simulink model "Three_ph_VSI_R2017a"  (R2020b)
settings: Solver=ode23tb  StartTime=0.0  StopTime=0.5  MaxStep=1e-6  RelTol=1e-3  EnableMultiTasking=on
libraries: powerlib x16, simulink x1
settings Model: Creator=shaheb  LastModifiedBy=HP
settings DataIOCC: LimitDataPoints=on  SaveFormat=Array  SignalLoggingSaveFormat=ModelDataLogs  ReturnWorkspaceOutputs=off
settings OptimizationCC: ExpressionDepthLimit=2147483647  LifeSpan=inf
settings DebuggingCC: UnderspecifiedInitializationDetection=Classic  MergeDetectMultiDrivingBlocksExec=none  SolverPrmCheckMsg=warning  FcnCallInpInsideContextMsg=warning  StateNameClashWarn=warning  SFUnexpectedBacktrackingDiag=warning  SFNoUnconditionalDefaultTransitionDiag=warning  ArithmeticOperatorsInVariantConditions=warning
settings HardwareCC: ProdBitPerPointer=32  ProdBitPerSizeT=32  ProdBitPerPtrDiffT=32  ProdLargestAtomicFloat=None  ProdIntDivRoundTo=Undefined  ProdEndianess=Unspecified  ProdWordSize=32  ProdHWDeviceType=32-bit Generic
settings ModelReferenceCC: PropagateSignalLabelsOutOfModel=off
settings SFSimCC: SimUseLocalCustomCode=off  CustomCodeUndefinedFunction=UseInterfaceOnly
settings RTWCC: RTWUseLocalCustomCode=off
settings CodeAppCC: StateflowObjectComments=on
settings GRTTargetCC: TargetLangStandard=C89/C90 (ANSI)  CombineOutputUpdateFcns=off  GRTInterface=on
settings ConfigComp: CovMetricSettings=dw  CovSaveCumulativeToWorkspaceVar=on  CovSaveSingleToWorkspaceVar=on  CovExternalEMLEnable=off
settings SimscapeCC: SimscapeNormalizeSystem=off

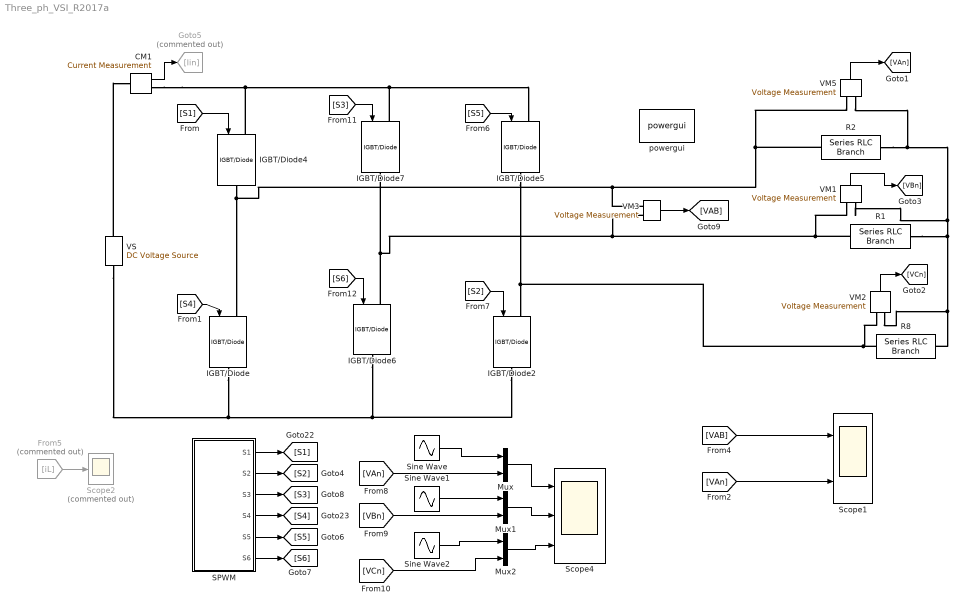
== system Three_ph_VSI_R2017a ==
  CM1 : powerlib/Measurements/Current Measurement  PhasorSimulation=off  OutputType=Complex  PSBequivalent=0
  From5 : From  Commented=on  GotoTag=iL
  Goto5 : Goto  Commented=on  GotoTag=Iin
  IGBT/Diode{,2,4..7} (6 alike) : powerlib/Power Electronics/IGBT//Diode  Ron=20e-3  Rs=1e5  Cs=inf  Measurements=off
  Mux : Mux  Inputs=2
  Mux1 : Mux  Inputs=2
  Mux2 : Mux  Inputs=2
  R1 : powerlib/Elements/Series RLC Branch  LConnTagsString=__new0  RConnTagsString=__new0  BranchType=RL  Resistance=40  Inductance=20e-3  SetiL0=off  InitialCurrent=0  Capacitance=500e-6  Setx0=off  InitialVoltage=0  Measurements=None
  R2 : powerlib/Elements/Series RLC Branch  LConnTagsString=__new0  RConnTagsString=__new0  BranchType=RL  Resistance=40  Inductance=20e-3  SetiL0=off  InitialCurrent=0  Capacitance=500e-6  Setx0=off  InitialVoltage=0  Measurements=None
  R8 : powerlib/Elements/Series RLC Branch  LConnTagsString=__new0  RConnTagsString=__new0  BranchType=RL  Resistance=40  Inductance=20e-3  SetiL0=off  InitialCurrent=0  Capacitance=500e-6  Setx0=off  InitialVoltage=0  Measurements=None
  SPWM : Subsystem
  Scope1 : Scope  NumInputPorts=2
  Scope2 : Scope  Commented=on
  Scope4 : Scope  NumInputPorts=3
  Sine Wave : Sin  Amplitude=230*sqrt(2)  Frequency=2*pi*50  SampleTime=0
  Sine Wave1 : Sin  Amplitude=230*sqrt(2)  Frequency=2*pi*50  Phase=-(2*pi/3)  SampleTime=0
  Sine Wave2 : Sin  Amplitude=230*sqrt(2)  Frequency=2*pi*50  Phase=+(2*pi/3)  SampleTime=0
  VM{1..3,5} (4 alike) : powerlib/Measurements/Voltage Measurement  PhasorSimulation=off  OutputType=Complex  PSBequivalent=0
  VS : powerlib/Electrical Sources/DC Voltage Source  Amplitude=700  Measurements=None
  powergui : powerlib/powergui  Priority=1  SimulationMode=Discrete  SampleTime=1e-6  frequency=60  Iterations=50  frequencyindice=0  Pbase=100e6  ErrMax=1e-4  UnitsV=kV  UnitsW=MW  buscounter=0  FunctionMessages=off  echomessages=off  EnableUseOfTLC=off  CurrentSourceSwitches=off  DisableSnubberDevices=off  DisableRonSwitches=off  DisableVfSwitches=off  DisplayEquations=off  AutomaticDiscreteSolvers=off  SolverType=Tustin  Interpol=off  ExternalGateDelay=off  methode=off  Ts=10  x0status=blocks  SPID=off  SwTol=0  HookPort=off  NonlinearTolerance=1e-4  nMaxIteration=100  ContinueOnMaxIteration=off  RestoreLinks=warning  ResistiveCurrentMeasurement=off  Frange=[0:2:500]  Ylog=off  Xlog=on  ShowGrid=off  save=off  variable=ZData  structure=vo  ZoomFFT=off  StartTime=0.2  cycles=10  DisplayStyle=1  fundamental=50  FreqAxis=on  MaxFrequency=20000  frequencyindicesteady=1  RmsSteady=1  display=off
  wires:
  [VAB] -> Scope1/1
  From5/1 -> Scope2/1
  SPWM/1(S1) -> [S1]
  SPWM/4(S4) -> [S4]
  VM2/1 -> [VCn]
  SPWM/6(S6) -> [S6]
  SPWM/5(S5) -> [S5]
  SPWM/3(S3) -> [S3]
  SPWM/2(S2) -> [S2]
  Sine Wave/1 -> Mux/1
  [VAn] -> Mux/2
  Mux/1 -> Scope4/1
  Sine Wave1/1 -> Mux1/1
  [VBn] -> Mux1/2
  Mux1/1 -> Scope4/2
  Sine Wave2/1 -> Mux2/1
  [VCn] -> Mux2/2
  Mux2/1 -> Scope4/3
  [S1] -> IGBT/Diode4/1
  [S4] -> IGBT/Diode/1
  CM1/1 -> Goto5/1
  [S5] -> IGBT/Diode5/1
  [S2] -> IGBT/Diode2/1
  [S3] -> IGBT/Diode7/1
  [S6] -> IGBT/Diode6/1
  VM5/1 -> [VAn]
  VM1/1 -> [VBn]
  VM3/1 -> [VAB]
  [VAn] -> Scope1/2
  connections:
  R2/LConn1 -- VM1/LConn2 -- R1/LConn1 -- VM2/LConn2 -- R8/LConn1 -- VM5/LConn2
  CM1/RConn1 -- IGBT/Diode4/LConn1 -- IGBT/Diode7/LConn1 -- IGBT/Diode5/LConn1
  IGBT/Diode7/RConn1 -- VM3/LConn2 -- R1/RConn1 -- VM1/LConn1 -- IGBT/Diode6/LConn1
  VS/LConn1 -- IGBT/Diode2/RConn1 -- IGBT/Diode6/RConn1 -- IGBT/Diode/RConn1
  IGBT/Diode4/RConn1 -- VM5/LConn1 -- R2/RConn1 -- VM3/LConn1 -- IGBT/Diode/LConn1
  IGBT/Diode5/RConn1 -- VM2/LConn1 -- R8/RConn1 -- IGBT/Diode2/LConn1
  VS/RConn1 -- CM1/LConn1

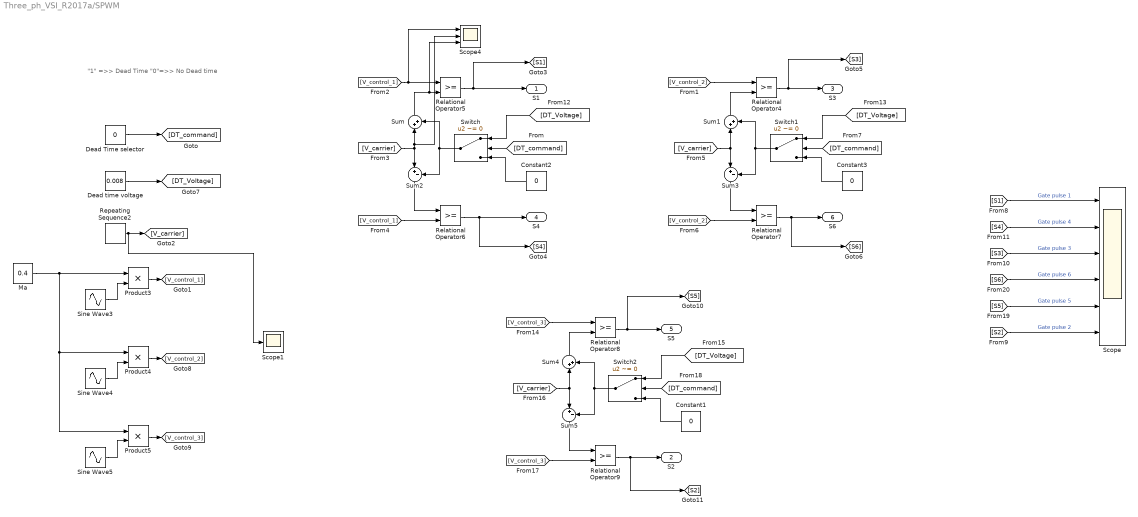
== system Three_ph_VSI_R2017a/SPWM ==
  note: "1" =>> Dead Time
      | "0"=>> No Dead time
  Constant1 : Constant  Value=0
  Constant2 : Constant  Value=0
  Constant3 : Constant  Value=0
  Dead Time selector : Constant  Value=0
  Dead time voltage : Constant  Value=0.008
  Ma : Constant  Value=0.4
  Product3 : Product
  Product4 : Product
  Product5 : Product
  Relational Operator{4..9} (6 alike) : RelationalOperator  OutDataTypeStr=boolean  RndMeth=Nearest
  Repeating Sequence2 : simulink/Sources/Repeating Sequence  rep_seq_t=[0 1/4 1/2 3/4 1/1]*1/(15*1000)  rep_seq_y=[0 1 0 -1 0]
  Scope : Scope  NumInputPorts=6
  Scope1 : Scope
  Scope4 : Scope  NumInputPorts=3
  Sine Wave3 : Sin  Frequency=2*pi*50  SampleTime=0
  Sine Wave4 : Sin  Frequency=2*pi*50  Phase=-(2*pi/3)  SampleTime=0
  Sine Wave5 : Sin  Frequency=2*pi*50  Phase=+(2*pi/3)  SampleTime=0
  Sum : Sum  Inputs=|++
  Sum1 : Sum  Inputs=|++
  Sum2 : Sum  Inputs=|+-
  Sum3 : Sum  Inputs=|+-
  Sum4 : Sum  Inputs=|++
  Sum5 : Sum  Inputs=|+-
  Switch : Switch  Criteria=u2 ~= 0
  Switch1 : Switch  Criteria=u2 ~= 0
  Switch2 : Switch  Criteria=u2 ~= 0
  S1 : Outport
  S2 : Outport  Port=2
  S3 : Outport  Port=3
  S4 : Outport  Port=4
  S5 : Outport  Port=5
  S6 : Outport  Port=6
  wires:
  Relational Operator6/1 -> S4/1, [S4]
  Constant2/1 -> Switch/3
  [V_control_1] -> Scope4/1, Relational Operator5/1
  Sum/1 -> Scope4/3, Relational Operator5/2
  [V_carrier] -> Scope4/2, Sum/1, Sum2/1
  Sine Wave3/1 -> Product3/2
  Dead time voltage/1 -> [DT_Voltage]
  Relational Operator5/1 -> [S1], S1/1
  [DT_Voltage] -> Switch/1
  Relational Operator4/1 -> S3/1, [S3]
  Switch1/1 -> Sum3/2, Sum1/2
  [DT_command] -> Switch/2
  Dead Time selector/1 -> [DT_command]
  [V_control_1] -> Relational Operator6/2
  [V_control_2] -> Relational Operator4/1
  Switch/1 -> Sum2/2, Sum/2
  Sum1/1 -> Relational Operator4/2
  Relational Operator7/1 -> [S6], S6/1
  Sum2/1 -> Relational Operator6/1
  [V_control_2] -> Relational Operator7/2
  [V_carrier] -> Sum3/1, Sum1/1
  [DT_command] -> Switch1/2
  [S6] -> Scope/4  "Gate pulse 6"
  Sum3/1 -> Relational Operator7/1
  [S4] -> Scope/2  "Gate pulse 4"
  Constant3/1 -> Switch1/3
  [DT_Voltage] -> Switch1/1
  [S3] -> Scope/3  "Gate pulse 3"
  [S1] -> Scope/1  "Gate pulse 1"
  Product3/1 -> [V_control_1]
  Product4/1 -> [V_control_2]
  Sine Wave4/1 -> Product4/2
  Sine Wave5/1 -> Product5/2
  Product5/1 -> [V_control_3]
  Ma/1 -> Product5/1, Product4/1, Product3/1
  [DT_Voltage] -> Switch2/1
  Constant1/1 -> Switch2/3
  Sum5/1 -> Relational Operator9/1
  [DT_command] -> Switch2/2
  [V_carrier] -> Sum4/1, Sum5/1
  [V_control_3] -> Relational Operator9/2
  Relational Operator9/1 -> S2/1, [S2]
  Sum4/1 -> Relational Operator8/2
  [V_control_3] -> Relational Operator8/1
  Switch2/1 -> Sum4/2, Sum5/2
  Relational Operator8/1 -> S5/1, [S5]
  [S2] -> Scope/6  "Gate pulse 2"
  [S5] -> Scope/5  "Gate pulse 5"
  Repeating Sequence2/1 -> Scope1/1, [V_carrier]
